simulink model "house_with_pid"  (R2020b)
settings: Solver=ode45  StartTime=0.0  StopTime=4*3600  RelTol=1e-3  EnableMultiTasking=on
undefined symbols (not defined in the file): C_R, K, Q_F_ON, Q_H, t_a, t_init, t_R_set, tau_F, tau_s
libraries: pid_lib x1, simulink_extras x1
settings Model: Creator=sgt  LastModifiedBy=Hammer
settings DataIOCC: LimitDataPoints=on  SaveFormat=Array  SignalLoggingSaveFormat=ModelDataLogs
settings OptimizationCC: ExpressionDepthLimit=2147483647  InitFltsAndDblsToZero=on  LifeSpan=inf
settings DebuggingCC: SaveWithParameterizedLinksMsg=none  UnderspecifiedInitializationDetection=Classic  MergeDetectMultiDrivingBlocksExec=none  SignalResolutionControl=TryResolveAllWithWarning  SolverPrmCheckMsg=warning  MultiTaskDSMMsg=warning  MultiTaskCondExecSysMsg=none  StateNameClashWarn=warning  SFUnexpectedBacktrackingDiag=warning  SFNoUnconditionalDefaultTransitionDiag=warning  SFExecutionAtInitializationDiag=none  ArithmeticOperatorsInVariantConditions=warning
settings HardwareCC: ProdBitPerPointer=32  ProdBitPerSizeT=32  ProdBitPerPtrDiffT=32  ProdLargestAtomicFloat=None  ProdIntDivRoundTo=Undefined  ProdEndianess=Unspecified  ProdWordSize=32  ProdHWDeviceType=32-bit Generic
settings ModelReferenceCC: PropagateSignalLabelsOutOfModel=off
settings SFSimCC: SimUseLocalCustomCode=off  CustomCodeUndefinedFunction=UseInterfaceOnly
settings RTWCC: RTWUseLocalCustomCode=off
settings CodeAppCC: StateflowObjectComments=on
settings GRTTargetCC: TargetFcnLib=ansi_tfl_tmw.mat  TargetLangStandard=C89/C90 (ANSI)  CombineOutputUpdateFcns=off  GRTInterface=on
settings ConfigComp: CovMetricSettings=dw  CovSaveCumulativeToWorkspaceVar=on  CovSaveSingleToWorkspaceVar=on  CovExternalEMLEnable=off  CovSFcnEnable=off

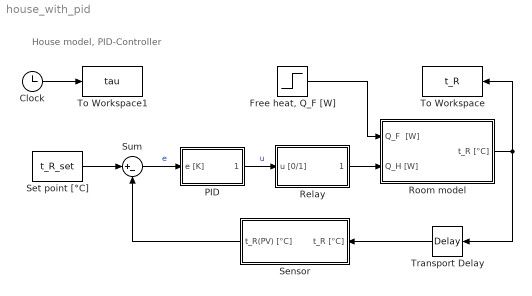
== system house_with_pid ==
  note: House model, PID-Controller
  Clock : Clock
  "Free heat, Q_F [W]" : Step  Time=tau_F  After=Q_F_ON  SampleTime=0
  PID : Subsystem
  Relay : Subsystem
  Room model : Subsystem
  Sensor : Subsystem
  Set point [°C] : Constant  Value=t_R_set
  Sum : Sum  Inputs=|+-
  To Workspace : ToWorkspace  VariableName=t_R  SampleTime=-1
  To Workspace1 : ToWorkspace  VariableName=tau  SampleTime=-1
  Transport Delay : TransportDelay  DelayTime=0
  wires:
  Clock/1 -> To Workspace1/1
  "Free heat, Q_F [W]"/1 -> Room model/1(Q_F  [W])
  Room model/1(t_R [°C]) -> To Workspace/1, Transport Delay/1
  Relay/1(Q_H [W]) -> Room model/2(Q_H [W])
  PID/1(u [0/1]) -> Relay/1(u [0/1])  "u"
  Set point [°C]/1 -> Sum/1
  Sensor/1(t_R(PV) [°C]) -> Sum/2
  Sum/1 -> PID/1(e [K])  "e"
  Transport Delay/1 -> Sensor/1(t_R [°C])

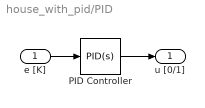
== system house_with_pid/PID ==
  e [K] : Inport
  PID Controller : pid_lib/PID Controller  Controller=PID  Form=Parallel  TimeDomain=Continuous-time  UseExternalTs=off  SampleTime=-1  IntegratorMethod=Forward Euler  FilterMethod=Forward Euler  ControllerParametersSource=internal  P=1.31115869505421  I=0.00102007570773898  D=45.1755961232093  UseFilter=on  N=0.0473242120593545  TunerSelectOption=Transfer Function Based (PID Tuner App)  InitialConditionSource=internal  InitialConditionForIntegrator=0  InitialConditionForFilter=0  DifferentiatorICPrevScaledInput=0  ExternalReset=none  TrackingMode=off  Kt=1  LimitOutput=off  SatLimitsSource=internal  UpperSaturationLimit=inf  LowerSaturationLimit=-inf  LinearizeAsGain=on  AntiWindupMode=none  Kb=1  POutMin=[]  POutMax=[]  IOutMin=[]  IOutMax=[]  DOutMin=[]  DOutMax=[]  NOutMin=[]  NOutMax=[]  SumOutMin=[]  SumOutMax=[]  SaturationOutMin=[]  SaturationOutMax=[]  PParamMin=[]  PParamMax=[]  IParamMin=[]  IParamMax=[]  DParamMin=[]  DParamMax=[]  NParamMin=[]  NParamMax=[]  KbParamMin=[]  KbParamMax=[]  KtParamMin=[]  KtParamMax=[]  KbOutMin=[]  KbOutMax=[]  KtOutMin=[]  KtOutMax=[]  IntegratorOutMin=[]  IntegratorOutMax=[]  FilterOutMin=[]  FilterOutMax=[]  SumI1OutMin=[]  SumI1OutMax=[]  SumI2OutMin=[]  SumI2OutMax=[]  SumI3OutMin=[]  SumI3OutMax=[]  SumI4OutMin=[]  SumI4OutMax=[]  SumDOutMin=[]  SumDOutMax=[]  DifferentiatorOutMin=[]  DifferentiatorOutMax=[]  FilterDiffOutCoefMin=[]  FilterDiffOutCoefMax=[]  ReciprocalOutMin=[]  ReciprocalOutMax=[]  SumDenOutMin=[]  SumDenOutMax=[]  SumNumOutMin=[]  SumNumOutMax=[]  DivideOutMin=[]  DivideOutMax=[]  UdiffTsProdOutMin=[]  UdiffTsProdOutMax=[]  NTsProdOutMin=[]  NTsProdOutMax=[]  UintegralTsProdOutMin=[]  UintegralTsProdOutMax=[]  UngainTsProdOutMin=[]  UngainTsProdOutMax=[]  IntegratorContinuousStateAttributes=''  IntegratorStateMustResolveToSignalObject=off  IntegratorRTWStateStorageClass=Auto  FilterContinuousStateAttributes=''  FilterStateMustResolveToSignalObject=off  FilterRTWStateStorageClass=Auto  ParallelPVariant=InternalParameters  IdealPVariant=Disabled  IVariant=InternalParameters  DVariant=InternalParameters  IntegratorVariant=Continuous  SatVariant=Disabled  AWVariant=Passthrough  PCopyVariant=Disabled  TRVariant=Disabled  FdbkBlocksVariant=Forward  IdealPFdbkVariant=Disabled  SatFdbkVariant=Disabled  DerivativeFilterVariant=ContFilter  NVariant=InternalParameters  NCopyVariant=Disabled  FilterICVariant=InternalICsFilter  IntegratorICVariant=InternalICs  ExternalResetVariant=Disabled  TRSumVariant=Passthrough  SumFdbkVariant=Disabled  SumVariant=Sum_PID  TsampFilterVariant=InternalTs  TsampNgainVariant=Passthrough  TsampIntegralVariant=Passthrough  ExternalSaturationOutDataTypeStr=Inherit: Same as second input
  u [0/1] : Outport
  wires:
  e [K]/1 -> PID Controller/1
  PID Controller/1 -> u [0/1]/1

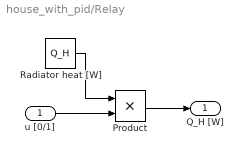
== system house_with_pid/Relay ==
  u [0/1] : Inport
  Product : Product  RndMeth=Zero
  Radiator heat [W] : Constant  Value=Q_H
  Q_H [W] : Outport
  wires:
  Radiator heat [W]/1 -> Product/1
  Product/1 -> Q_H [W]/1
  u [0/1]/1 -> Product/2

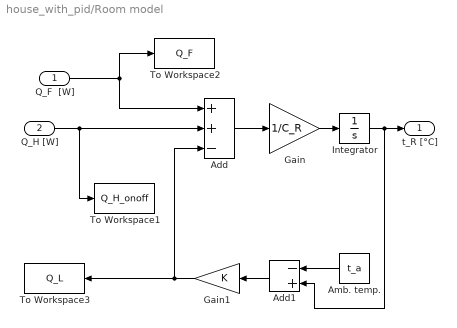
== system house_with_pid/Room model ==
  Q_F  [W] : Inport
  Q_H [W] : Inport  Port=2
  Add : Sum  Inputs=++-
  Add1 : Sum  Inputs=-+
  Amb. temp. : Constant  Value=t_a
  Gain : Gain  Gain=1/C_R
  Gain1 : Gain  Gain=K
  Integrator : Integrator  InitialCondition=t_init
  To Workspace1 : ToWorkspace  VariableName=Q_H_onoff  SampleTime=-1
  To Workspace2 : ToWorkspace  VariableName=Q_F  SampleTime=-1
  To Workspace3 : ToWorkspace  VariableName=Q_L  SampleTime=-1
  t_R [°C] : Outport
  wires:
  Integrator/1 -> Add1/2, t_R [°C]/1
  Gain/1 -> Integrator/1
  Add/1 -> Gain/1
  Q_F  [W]/1 -> To Workspace2/1, Add/1
  Amb. temp./1 -> Add1/1
  Add1/1 -> Gain1/1
  Gain1/1 -> Add/3, To Workspace3/1
  Q_H [W]/1 -> Add/2, To Workspace1/1

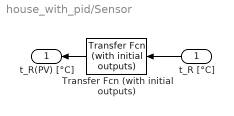
== system house_with_pid/Sensor ==
  t_R [°C] : Inport
  Transfer Fcn (with initial outputs) : simulink_extras/Additional Linear/Transfer Fcn (with initial outputs)  N=[1]  D="[tau_s  1]"  Y0=t_init  U0=0
  t_R(PV) [°C] : Outport
  wires:
  t_R [°C]/1 -> Transfer Fcn (with initial outputs)/1
  Transfer Fcn (with initial outputs)/1 -> t_R(PV) [°C]/1
